simulink model "RadarSimulinkProjectRev009"  (R2024a)
settings: Solver=VariableStepAuto  StartTime=0.0  StopTime=0.0125  RelTol=1e-3
values from neighbouring files (symbols this model uses):
  AngleTime = SweepTime/10    (= 10000)    [InitializationOfVariables.m]    (also in InitializationOfVariablesRev000.m; InitializationOfVariablesRev001.m; InitializationOfVariablesRev003.m = 2097152; InitializationOfVariablesRev004.m = 2097152)
  ASR_LUT = Rsamp-OffsetDelayR    [InitializationOfVariablesRev003.m]    (also in InitializationOfVariablesRev004.m = round((R*2*SystemFs)/c))
  Btn_Debounce = 20000    [InitializationOfVariablesRev003.m]    (also in InitializationOfVariablesRev004.m)
  ChirpNc = 128    [InitializationOfVariablesRev003.m]    (also in InitializationOfVariablesRev004.m)
  ChirpSizeLength = FreqDeltaPeriod*361    (= 16245)    [InitializationOfVariablesRev003.m]    (also in InitializationOfVariablesRev004.m = 16384)
  DeciFactor = 8    [InitializationOfVariablesRev004.m]
  FCW = [FCW_p1, FCW_p2]    [InitializationOfVariablesRev003.m]    (also in InitializationOfVariablesRev004.m = f / SystemFs)
  RXFFTLength = 16384    [InitializationOfVariablesRev003.m]    (also in InitializationOfVariablesRev004.m = 2048)
  SweepTime = 100000    [InitializationOfVariables.m]    (also in InitializationOfVariablesRev000.m; InitializationOfVariablesRev001.m; InitializationOfVariablesRev003.m = 23068672; InitializationOfVariablesRev004.m = 23068672)
undefined symbols (not defined in the file or in its folder): SignalGenerationForAnalysis, Subsystem, xc7a200tfbg676
libraries: hdlBasic x407, hdlUtilities x11, hdlDSPIP x11, vmcUtilities x1
(part 3 of 4)

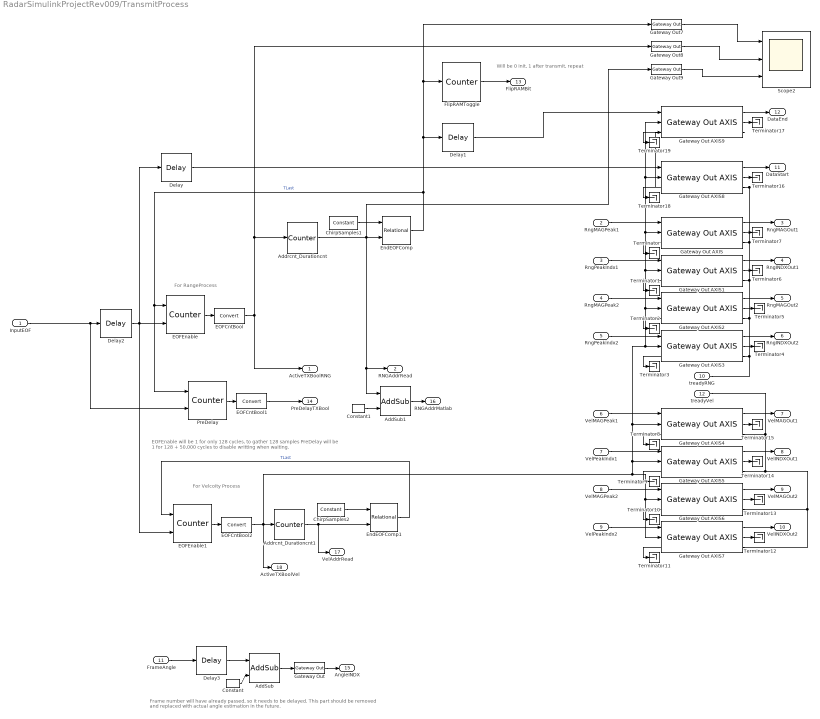
== system RadarSimulinkProjectRev009/TransmitProcess ==
  note: For RangeProcess
  note: Frame number will have already passed, so it needs to be delayed. This part should be removed and replaced with actual angle estimation in the future.
  note: EOFEnable will be 1 for only 128 cycles, to gather 128 samples
      | PreDelay will be 1 for 128 + 50,000 cycles to disable writting when waiting.
  note: Will be 0 init, 1 after transmit, repeat
  note: For Velcoity Process
  InputEOF : Inport
  RngMAGPeak1 : Inport  Port=2
  RngPeakIndx1 : Inport  Port=3
  RngMAGPeak2 : Inport  Port=4
  RngPeakindx2 : Inport  Port=5
  VelMAGPeak1 : Inport  Port=6
  VelPeakIndx1 : Inport  Port=7
  VelMAGPeak2 : Inport  Port=8
  VelPeakindx2 : Inport  Port=9
  treadyRNG : Inport  Port=10
  FrameAngle : Inport  Port=11
  treadyVel : Inport  Port=12
  AddSub : hdlBasic/AddSub  mode=Addition  use_carryin=off  use_carryout=off  en=off  latency=1  precision=Full  arith_type=Unsigned  n_bits=16  bin_pt=14  quantization=Truncate  overflow=Wrap  use_behavioral_HDL=off  hw_selection=Fabric  pipelined=off  XmcBlockStatus=1  maskContainerNames=tabcontainer1  block_type=addsub  block_config=sysgen:Addsub_config
  AddSub1 : hdlBasic/AddSub  mode=Addition  use_carryin=off  use_carryout=off  en=off  latency=1  precision=Full  arith_type=Unsigned  n_bits=16  bin_pt=14  quantization=Truncate  overflow=Wrap  use_behavioral_HDL=off  hw_selection=Fabric  pipelined=off  XmcBlockStatus=1  maskContainerNames=tabcontainer1  block_type=addsub  block_config=sysgen:Addsub_config
  Addrcnt_Durationcnt : hdlBasic/Counter  cnt_type=Count limited  cnt_to=ChirpNc-1  operation=Up  start_count=0  cnt_by_val=1  arith_type=Unsigned  n_bits=7  bin_pt=0  load_pin=off  rst=off  en=on  explicit_period=Explicit  period=P1  use_behavioral_HDL=off  implementation=Fabric  XmcBlockStatus=1  maskContainerNames=group1  block_type=counter  block_config=sysgen:Counter_config  block_width=531  block_height=1023
  Addrcnt_Durationcnt1 : hdlBasic/Counter  cnt_type=Count limited  cnt_to=RXFFTLength-1  operation=Up  start_count=0  cnt_by_val=1  arith_type=Unsigned  n_bits=11  bin_pt=0  load_pin=off  rst=off  en=on  explicit_period=Explicit  period=P1  use_behavioral_HDL=off  implementation=Fabric  XmcBlockStatus=1  maskContainerNames=group1  block_type=counter  block_config=sysgen:Counter_config  block_width=531  block_height=1023
  ChirpSamples1 : hdlBasic/Constant  const=127  gui_display_data_type=Fixed-point  arith_type=Unsigned  n_bits=7  bin_pt=0  preci_type=Single  exp_width=8  frac_width=24  explicit_period=on  period=P2  XmcBlockStatus=1  maskContainerNames=tabcontainer1  block_type=constant  block_config=sysgen:Constant_config
  ChirpSamples2 : hdlBasic/Constant  const=2047  gui_display_data_type=Fixed-point  arith_type=Unsigned  n_bits=15  bin_pt=0  preci_type=Single  exp_width=8  frac_width=24  explicit_period=on  period=P2  XmcBlockStatus=1  maskContainerNames=tabcontainer1  block_type=constant  block_config=sysgen:Constant_config
  Constant : hdlBasic/Constant  const=1.0  gui_display_data_type=Fixed-point  arith_type=Unsigned  n_bits=7  bin_pt=0  preci_type=Single  exp_width=8  frac_width=24  explicit_period=off  period=1  XmcBlockStatus=1  maskContainerNames=tabcontainer1  block_type=constant  block_config=sysgen:Constant_config
  Constant1 : hdlBasic/Constant  const=1.0  gui_display_data_type=Fixed-point  arith_type=Unsigned  n_bits=7  bin_pt=0  preci_type=Single  exp_width=8  frac_width=24  explicit_period=off  period=1  XmcBlockStatus=1  maskContainerNames=tabcontainer1  block_type=constant  block_config=sysgen:Constant_config
  Delay : hdlBasic/Delay  rst=off  en=off  latency=1  reg_retiming=off  XmcBlockStatus=1  maskContainerNames=group1  block_type=delay  block_config=sysgen:Delay_config
  Delay1 : hdlBasic/Delay  rst=off  en=off  latency=1  reg_retiming=off  XmcBlockStatus=1  maskContainerNames=group1  block_type=delay  block_config=sysgen:Delay_config
  Delay2 : hdlBasic/Delay  rst=off  en=off  latency=50000  reg_retiming=off  XmcBlockStatus=1  maskContainerNames=group1  block_type=delay  block_config=sysgen:Delay_config
  Delay3 : hdlBasic/Delay  rst=off  en=off  latency=64000  reg_retiming=off  XmcBlockStatus=1  maskContainerNames=group1  block_type=delay  block_config=sysgen:Delay_config
  EOFCntBool : hdlBasic/Convert  gui_display_data_type=Boolean  arith_type=Boolean  n_bits=16  bin_pt=14  float_type=Single  exp_bits=8  fraction_bits=24  quantization=Truncate  overflow=Wrap  en=off  latency=0  pipeline=off  XmcBlockStatus=1  maskContainerNames=group2  block_type=convert  block_config=sysgen:Convert_config  block_width=595  block_height=885
  EOFCntBool1 : hdlBasic/Convert  gui_display_data_type=Boolean  arith_type=Boolean  n_bits=16  bin_pt=14  float_type=Single  exp_bits=8  fraction_bits=24  quantization=Truncate  overflow=Wrap  en=off  latency=0  pipeline=off  XmcBlockStatus=1  maskContainerNames=group2  block_type=convert  block_config=sysgen:Convert_config  block_width=595  block_height=885
  EOFCntBool2 : hdlBasic/Convert  gui_display_data_type=Boolean  arith_type=Boolean  n_bits=16  bin_pt=14  float_type=Single  exp_bits=8  fraction_bits=24  quantization=Truncate  overflow=Wrap  en=off  latency=0  pipeline=off  XmcBlockStatus=1  maskContainerNames=group2  block_type=convert  block_config=sysgen:Convert_config  block_width=595  block_height=885
  EOFEnable : hdlBasic/Counter  cnt_type=Count limited  cnt_to=1  operation=Up  start_count=0  cnt_by_val=1  arith_type=Unsigned  n_bits=1  bin_pt=0  load_pin=off  rst=on  en=on  explicit_period=Explicit  period=P1  use_behavioral_HDL=off  implementation=Fabric  XmcBlockStatus=1  maskContainerNames=group1  block_type=counter  block_config=sysgen:Counter_config  block_width=531  block_height=1023
  EOFEnable1 : hdlBasic/Counter  cnt_type=Count limited  cnt_to=1  operation=Up  start_count=0  cnt_by_val=1  arith_type=Unsigned  n_bits=1  bin_pt=0  load_pin=off  rst=on  en=on  explicit_period=Explicit  period=P1  use_behavioral_HDL=off  implementation=Fabric  XmcBlockStatus=1  maskContainerNames=group1  block_type=counter  block_config=sysgen:Counter_config  block_width=531  block_height=1023
  EndEOFComp : hdlBasic/Relational  mode=a=b  op_type=Bool  en=off  latency=0  XmcBlockStatus=1  maskContainerNames=tabcontainer1  block_type=relational  block_config=sysgen:Relational_config
  EndEOFComp1 : hdlBasic/Relational  mode=a=b  op_type=Bool  en=off  latency=0  XmcBlockStatus=1  maskContainerNames=tabcontainer1  block_type=relational  block_config=sysgen:Relational_config
  FlipRAMToggle : hdlBasic/Counter  cnt_type=Count limited  cnt_to=1  operation=Up  start_count=0  cnt_by_val=1  arith_type=Unsigned  n_bits=1  bin_pt=0  load_pin=off  rst=off  en=on  explicit_period=Explicit  period=P1  use_behavioral_HDL=off  implementation=Fabric  XmcBlockStatus=1  maskContainerNames=group1  block_type=counter  block_config=sysgen:Counter_config  block_width=531  block_height=1023
  Gateway Out{,7..9} (4 alike) : hdlBasic/Gateway Out  inherit_from_input=off  bool_to_boolean=off  hdl_port=on  rows=1  columns=1  UseAsDAC=off  DACChannel='1'  interface=None  automatic_assignment=on  address_offset=hex2dec('00')  intf_name=''  intf_description=''  timing_constraint=None  locs_specified=off  LOCs={}  io_standard={}  XmcBlockStatus=1  maskContainerNames=group4  block_type=gatewayout  block_config=sysgen:gateway_out_config  block_width_w=590  block_height_w=620  block_width=620  block_height=750
  Gateway Out AXIS{,1..9} (10 alike) : hdlUtilities/Gateway Out AXIS  mask_sample_period=1  bool_to_boolean=off  block_type=gatewayoutaxi
  PreDelay : hdlBasic/Counter  cnt_type=Count limited  cnt_to=1  operation=Up  start_count=0  cnt_by_val=1  arith_type=Unsigned  n_bits=1  bin_pt=0  load_pin=off  rst=on  en=on  explicit_period=Explicit  period=P1  use_behavioral_HDL=off  implementation=Fabric  XmcBlockStatus=1  maskContainerNames=group1  block_type=counter  block_config=sysgen:Counter_config  block_width=531  block_height=1023
  Scope2 : Scope  NumInputPorts=3
  Terminator{,1..19} (20 alike) : Terminator
  ActiveTXBoolRNG : Outport
  RNGAddrRead : Outport  Port=2
  RngMAGOut1 : Outport  Port=3
  RngINDXOut1 : Outport  Port=4
  RngMAGOut2 : Outport  Port=5
  RngINDXOut2 : Outport  Port=6
  VelMAGOut1 : Outport  Port=7
  VelINDXOut1 : Outport  Port=8
  VelMAGOut2 : Outport  Port=9
  VelINDXOut2 : Outport  Port=10
  DataStart : Outport  Port=11
  DataEnd : Outport  Port=12
  FlipRAMBit : Outport  Port=13
  PreDelayTXBool : Outport  Port=14
  AngleINDX : Outport  Port=15
  RNGAddrMatlab : Outport  Port=16
  VelAddrRead : Outport  Port=17
  ActiveTXBoolVel : Outport  Port=18
  wires:
  ChirpSamples1/1 -> EndEOFComp/1
  Gateway Out AXIS/1 -> RngMAGOut1/1
  Gateway Out AXIS2/3 -> Terminator2/1
  Gateway Out AXIS3/1 -> RngINDXOut2/1
  Gateway Out AXIS1/3 -> Terminator1/1
  Gateway Out AXIS1/1 -> RngINDXOut1/1
  Gateway Out AXIS/2 -> Terminator7/1
  EndEOFComp/1 -> Gateway Out7/1, FlipRAMToggle/1, Delay1/1, PreDelay/1, EOFEnable/1  "TLast"
  Gateway Out AXIS2/1 -> RngMAGOut2/1
  EOFEnable/1 -> EOFCntBool/1
  RngMAGPeak2/1 -> Gateway Out AXIS2/1
  Gateway Out AXIS2/2 -> Terminator5/1
  RngPeakIndx1/1 -> Gateway Out AXIS1/1
  RngMAGPeak1/1 -> Gateway Out AXIS/1
  Gateway Out AXIS1/2 -> Terminator6/1
  RngPeakindx2/1 -> Gateway Out AXIS3/1
  Gateway Out AXIS3/3 -> Terminator3/1
  Gateway Out AXIS3/2 -> Terminator4/1
  Gateway Out AXIS/3 -> Terminator/1
  Gateway Out AXIS7/3 -> Terminator11/1
  VelPeakindx2/1 -> Gateway Out AXIS7/1
  Gateway Out AXIS6/3 -> Terminator10/1
  VelMAGPeak2/1 -> Gateway Out AXIS6/1
  Gateway Out AXIS5/2 -> Terminator14/1
  Gateway Out AXIS6/1 -> VelMAGOut2/1
  Gateway Out AXIS7/1 -> VelINDXOut2/1
  Gateway Out AXIS5/1 -> VelINDXOut1/1
  EOFCntBool/1 -> Gateway Out8/1, Addrcnt_Durationcnt/1, ActiveTXBoolRNG/1
  VelPeakIndx1/1 -> Gateway Out AXIS5/1
  Gateway Out AXIS4/3 -> Terminator8/1
  Gateway Out AXIS6/2 -> Terminator13/1
  VelMAGPeak1/1 -> Gateway Out AXIS4/1
  Gateway Out AXIS7/2 -> Terminator12/1
  Gateway Out AXIS4/1 -> VelMAGOut1/1
  Gateway Out AXIS5/3 -> Terminator9/1
  Gateway Out AXIS4/2 -> Terminator15/1
  treadyRNG/1 -> Gateway Out AXIS9/3, Gateway Out AXIS8/3, Gateway Out AXIS/3, Gateway Out AXIS1/3, Gateway Out AXIS2/3, Gateway Out AXIS3/3
  Gateway Out AXIS8/1 -> DataStart/1
  Gateway Out AXIS8/2 -> Terminator16/1
  Gateway Out AXIS9/1 -> DataEnd/1
  Gateway Out AXIS9/2 -> Terminator17/1
  Gateway Out AXIS8/3 -> Terminator18/1
  Gateway Out AXIS9/3 -> Terminator19/1
  Delay/1 -> Gateway Out AXIS8/1
  Delay1/1 -> Gateway Out AXIS9/1
  Delay2/1 -> EOFEnable1/2, Delay/1, EOFEnable/2
  FlipRAMToggle/1 -> FlipRAMBit/1
  PreDelay/1 -> EOFCntBool1/1
  EOFCntBool1/1 -> PreDelayTXBool/1
  FrameAngle/1 -> Delay3/1
  Delay3/1 -> AddSub/1
  Gateway Out/1 -> AngleINDX/1
  Constant/1 -> AddSub/2
  AddSub/1 -> Gateway Out/1
  Addrcnt_Durationcnt/1 -> Gateway Out9/1, EndEOFComp/2, RNGAddrRead/1, AddSub1/1
  AddSub1/1 -> RNGAddrMatlab/1
  Constant1/1 -> AddSub1/2
  InputEOF/1 -> PreDelay/2, Delay2/1
  Addrcnt_Durationcnt1/1 -> VelAddrRead/1, EndEOFComp1/2
  ChirpSamples2/1 -> EndEOFComp1/1
  EndEOFComp1/1 -> EOFEnable1/1  "TLast"
  EOFEnable1/1 -> EOFCntBool2/1
  EOFCntBool2/1 -> ActiveTXBoolVel/1, Gateway Out AXIS4/2, Gateway Out AXIS3/2, Gateway Out AXIS9/2, Gateway Out AXIS8/2, Gateway Out AXIS/2, Gateway Out AXIS1/2, Gateway Out AXIS2/2, Gateway Out AXIS5/2, Gateway Out AXIS6/2, Gateway Out AXIS7/2, Addrcnt_Durationcnt1/1
  treadyVel/1 -> Gateway Out AXIS7/3, Gateway Out AXIS6/3, Gateway Out AXIS5/3, Gateway Out AXIS4/3
  Gateway Out8/1 -> Scope2/2
  Gateway Out9/1 -> Scope2/3
  Gateway Out7/1 -> Scope2/1

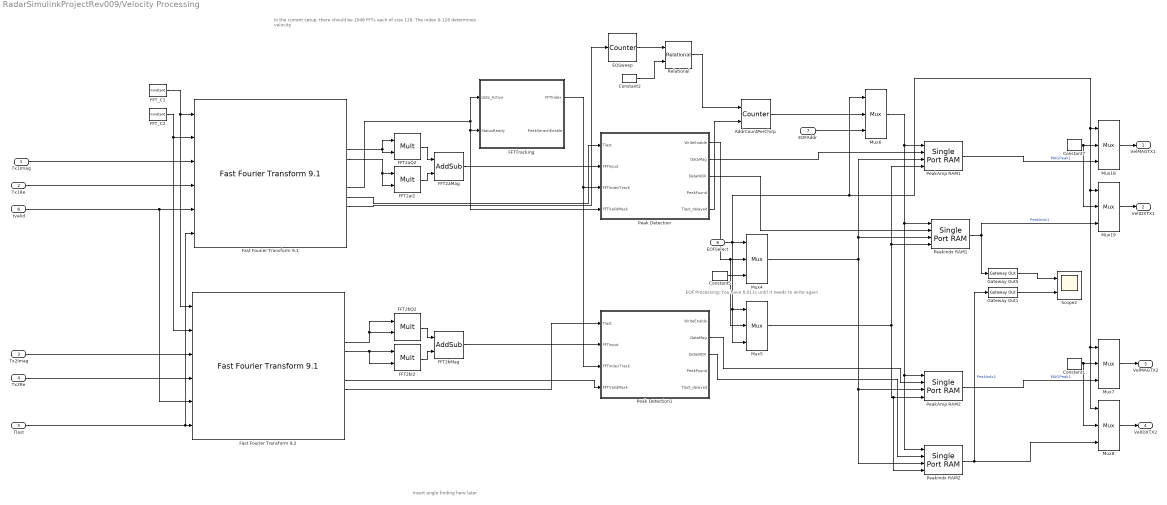
== system RadarSimulinkProjectRev009/Velocity Processing ==
  note: In the current setup, there should be 2048 FFTs each of size 128. The index 0-128 determines velocity
  note: EOF Processing: You have 0.011s until it needs to write again
  note: Insert angle finding here later
  Tx1Imag : Inport
  Tx1Re : Inport  Port=2
  Tx2Imag : Inport  Port=3
  Tx2Re : Inport  Port=4
  Tlast : Inport  Port=5
  tvalid : Inport  Port=6
  EOFAddr : Inport  Port=7
  EOFSelect : Inport  Port=8
  AddrCountPerChirp : hdlBasic/Counter  cnt_type=Count limited  cnt_to=RXFFTLength-1  operation=Up  start_count=0  cnt_by_val=1  arith_type=Unsigned  n_bits=11  bin_pt=0  load_pin=off  rst=on  en=on  explicit_period=Explicit  period=P1  use_behavioral_HDL=off  implementation=Fabric  XmcBlockStatus=1  maskContainerNames=group1  block_type=counter  block_config=sysgen:Counter_config  block_width=531  block_height=1023
  Constant1 : hdlBasic/Constant  const=0  gui_display_data_type=Fixed-point  arith_type=Signed (2's comp)  n_bits=16  bin_pt=15  preci_type=Single  exp_width=8  frac_width=24  explicit_period=on  period=P2  XmcBlockStatus=1  maskContainerNames=tabcontainer1  block_type=constant  block_config=sysgen:Constant_config
  Constant2 : hdlBasic/Constant  const=0  gui_display_data_type=Fixed-point  arith_type=Signed (2's comp)  n_bits=1  bin_pt=0  preci_type=Single  exp_width=8  frac_width=24  explicit_period=on  period=P1  XmcBlockStatus=1  maskContainerNames=tabcontainer1  block_type=constant  block_config=sysgen:Constant_config
  Constant5 : hdlBasic/Constant  const=0  gui_display_data_type=Boolean  arith_type=Boolean  n_bits=16  bin_pt=15  preci_type=Single  exp_width=8  frac_width=24  explicit_period=on  period=P2  XmcBlockStatus=1  maskContainerNames=tabcontainer1  block_type=constant  block_config=sysgen:Constant_config
  Constant7 : hdlBasic/Constant  const=0  gui_display_data_type=Fixed-point  arith_type=Signed (2's comp)  n_bits=16  bin_pt=15  preci_type=Single  exp_width=8  frac_width=24  explicit_period=on  period=P2  XmcBlockStatus=1  maskContainerNames=tabcontainer1  block_type=constant  block_config=sysgen:Constant_config
  EOSweep : hdlBasic/Counter  cnt_type=Count limited  cnt_to=ChirpNc*11-1  operation=Up  start_count=0  cnt_by_val=1  arith_type=Unsigned  n_bits=11  bin_pt=0  load_pin=off  rst=off  en=on  explicit_period=Explicit  period=P1  use_behavioral_HDL=off  implementation=Fabric  XmcBlockStatus=1  maskContainerNames=group1  block_type=counter  block_config=sysgen:Counter_config  block_width=531  block_height=1023
  FFT2aI2 : hdlBasic/Mult  precision=Full  arith_type="Signed  (2's comp)"  n_bits=16  bin_pt=14  quantization=Truncate  overflow=Wrap  en=off  latency=3  opt_float=off  fp_mult_usage=No Usage  use_behavioral_HDL=off  opt=Speed  use_embedded=on  optimum_pipeline=off  pipeline=on  use_rpm=on  placement_style=Triangular  XmcBlockStatus=1  maskContainerNames=group1  block_type=mult  block_config=sysgen:Mult_config  block_width=598  block_height=876
  FFT2aMag : hdlBasic/AddSub  mode=Addition  use_carryin=off  use_carryout=off  en=off  latency=0  precision=Full  arith_type=Unsigned  n_bits=16  bin_pt=14  quantization=Truncate  overflow=Wrap  use_behavioral_HDL=off  hw_selection=Fabric  pipelined=off  XmcBlockStatus=1  maskContainerNames=tabcontainer1  block_type=addsub  block_config=sysgen:Addsub_config
  FFT2aQ2 : hdlBasic/Mult  precision=Full  arith_type="Signed  (2's comp)"  n_bits=16  bin_pt=14  quantization=Truncate  overflow=Wrap  en=off  latency=3  opt_float=off  fp_mult_usage=No Usage  use_behavioral_HDL=off  opt=Speed  use_embedded=on  optimum_pipeline=off  pipeline=on  use_rpm=on  placement_style=Triangular  XmcBlockStatus=1  maskContainerNames=group1  block_type=mult  block_config=sysgen:Mult_config  block_width=598  block_height=876
  FFT2bI2 : hdlBasic/Mult  precision=Full  arith_type="Signed  (2's comp)"  n_bits=16  bin_pt=14  quantization=Truncate  overflow=Wrap  en=off  latency=3  opt_float=off  fp_mult_usage=No Usage  use_behavioral_HDL=off  opt=Speed  use_embedded=on  optimum_pipeline=off  pipeline=on  use_rpm=on  placement_style=Triangular  XmcBlockStatus=1  maskContainerNames=group1  block_type=mult  block_config=sysgen:Mult_config  block_width=598  block_height=876
  FFT2bMag : hdlBasic/AddSub  mode=Addition  use_carryin=off  use_carryout=off  en=off  latency=0  precision=Full  arith_type=Unsigned  n_bits=16  bin_pt=14  quantization=Truncate  overflow=Wrap  use_behavioral_HDL=off  hw_selection=Fabric  pipelined=off  XmcBlockStatus=1  maskContainerNames=tabcontainer1  block_type=addsub  block_config=sysgen:Addsub_config
  FFT2bQ2 : hdlBasic/Mult  precision=Full  arith_type="Signed  (2's comp)"  n_bits=16  bin_pt=14  quantization=Truncate  overflow=Wrap  en=off  latency=3  opt_float=off  fp_mult_usage=No Usage  use_behavioral_HDL=off  opt=Speed  use_embedded=on  optimum_pipeline=off  pipeline=on  use_rpm=on  placement_style=Triangular  XmcBlockStatus=1  maskContainerNames=group1  block_type=mult  block_config=sysgen:Mult_config  block_width=598  block_height=876
  FFTTracking : Subsystem
  FFT_C1 : hdlBasic/Constant  const=1.0  gui_display_data_type=Fixed-point  arith_type=Unsigned  n_bits=1  bin_pt=0  preci_type=Single  exp_width=8  frac_width=24  explicit_period=on  period=P2  XmcBlockStatus=1  maskContainerNames=tabcontainer1  block_type=constant  block_config=sysgen:Constant_config
  FFT_C2 : hdlBasic/Constant  const=1.0  gui_display_data_type=Boolean  arith_type=Boolean  n_bits=1  bin_pt=0  preci_type=Single  exp_width=8  frac_width=24  explicit_period=on  period=P2  XmcBlockStatus=1  maskContainerNames=tabcontainer1  block_type=constant  block_config=sysgen:Constant_config
  Fast Fourier Transform 9.1 : hdlDSPIP/Fast Fourier Transform 9.1   transform_length=128  target_clock_frequency=192  target_data_throughput=50  implementation_options=pipelined_streaming_io  run_time_configurable_transform_length=off  enable_ssr=off  super_sample_rates=1  data_format=fixed_point  phase_factor_width=32  scaling_options=block_floating_point  rounding_modes=truncation  aclken=off  aresetn=off  output_ordering=natural_order  cyclic_prefix_insertion=off  throttle_scheme=realtime  xk_index=on  ovflo=off  trim_axipin_name=on  memory_options_data=block_ram  memory_options_phase_factors=block_ram  number_of_stages_using_block_ram_for_data_and_phase_factors=2  memory_options_reorder=block_ram  memory_options_hybrid=off  complex_mult_type=use_mults_resources  butterfly_type=use_xtremedsp_slices  simulation_type=hybrid_sim  simulation_model=sysgen:xfftv9_cmodel  data_path_portlist={ 's_axis_data_tdata', 'm_axis_data_tdata', 'm_axis_status_tdata', 'event_fft_overflow' }  channels=1  input_ordering=natural_order  input_width=16  ip_name=Fast Fourier Transform  ip_version=9.1  dsptool_ready=true  ipcore_usecache=true  ipcore_useipmodelcache=true  wrapper_available=true  port_translation_map={ 'aclken' => 'en', 'aresetn' => 'rst'}  XmcBlockStatus=1  maskContainerNames=tabcontainer1  block_type=xfft_v9_1  block_config=sysgen:rodinimport_config
  Fast Fourier Transform 9.2 : hdlDSPIP/Fast Fourier Transform 9.1   transform_length=128  target_clock_frequency=192  target_data_throughput=50  implementation_options=pipelined_streaming_io  run_time_configurable_transform_length=off  enable_ssr=off  super_sample_rates=1  data_format=fixed_point  phase_factor_width=32  scaling_options=block_floating_point  rounding_modes=truncation  aclken=off  aresetn=off  output_ordering=natural_order  cyclic_prefix_insertion=off  throttle_scheme=realtime  xk_index=on  ovflo=off  trim_axipin_name=on  memory_options_data=block_ram  memory_options_phase_factors=block_ram  number_of_stages_using_block_ram_for_data_and_phase_factors=2  memory_options_reorder=block_ram  memory_options_hybrid=off  complex_mult_type=use_mults_resources  butterfly_type=use_xtremedsp_slices  simulation_type=hybrid_sim  simulation_model=sysgen:xfftv9_cmodel  data_path_portlist={ 's_axis_data_tdata', 'm_axis_data_tdata', 'm_axis_status_tdata', 'event_fft_overflow' }  channels=1  input_ordering=natural_order  input_width=16  ip_name=Fast Fourier Transform  ip_version=9.1  dsptool_ready=true  ipcore_usecache=true  ipcore_useipmodelcache=true  wrapper_available=true  port_translation_map={ 'aclken' => 'en', 'aresetn' => 'rst'}  XmcBlockStatus=1  maskContainerNames=tabcontainer1  block_type=xfft_v9_1  block_config=sysgen:rodinimport_config
  Gateway Out1 : hdlBasic/Gateway Out  inherit_from_input=off  bool_to_boolean=off  hdl_port=on  rows=1  columns=1  UseAsDAC=off  DACChannel='1'  interface=None  automatic_assignment=on  address_offset=hex2dec('00')  intf_name=''  intf_description=''  timing_constraint=None  locs_specified=off  LOCs={}  io_standard={}  XmcBlockStatus=1  maskContainerNames=group4  block_type=gatewayout  block_config=sysgen:gateway_out_config  block_width_w=590  block_height_w=620  block_width=620  block_height=750
  Gateway Out5 : hdlBasic/Gateway Out  inherit_from_input=off  bool_to_boolean=off  hdl_port=on  rows=1  columns=1  UseAsDAC=off  DACChannel='1'  interface=None  automatic_assignment=on  address_offset=hex2dec('00')  intf_name=''  intf_description=''  timing_constraint=None  locs_specified=off  LOCs={}  io_standard={}  XmcBlockStatus=1  maskContainerNames=group4  block_type=gatewayout  block_config=sysgen:gateway_out_config  block_width_w=590  block_height_w=620  block_width=620  block_height=750
  Mux{4..8,18..19} (7 alike) : hdlBasic/Mux  inputs=2  en=off  latency=0  precision=Full  arith_type=Unsigned  n_bits=16  bin_pt=14  quantization=Truncate  overflow=Wrap  XmcBlockStatus=1  maskContainerNames=tabcontainer1  block_type=mux  block_config=sysgen:Mux_config
  Peak Detection : Subsystem
  Peak Detection1 : Subsystem
  PeakAmp RAM1 : hdlBasic/Single Port RAM  depth=RXFFTLength  initVector=0  distributed_mem=Block RAM  write_mode=Read After Write  rst=off  init_reg=0  en=on  optimize_latency=off  latency=1  optimize=Area  dbl_ovrd=off  simulation_type=fast_sim  XmcBlockStatus=1  maskContainerNames=tabcontainer1  block_type=spram  block_config=sysgen:SPRAM_config
  PeakAmp RAM2 : hdlBasic/Single Port RAM  depth=RXFFTLength  initVector=0  distributed_mem=Block RAM  write_mode=Read After Write  rst=off  init_reg=0  en=on  optimize_latency=off  latency=1  optimize=Area  dbl_ovrd=off  simulation_type=fast_sim  XmcBlockStatus=1  maskContainerNames=tabcontainer1  block_type=spram  block_config=sysgen:SPRAM_config
  PeakIndx RAM1 : hdlBasic/Single Port RAM  depth=RXFFTLength  initVector=0  distributed_mem=Block RAM  write_mode=Read After Write  rst=off  init_reg=0  en=on  optimize_latency=off  latency=1  optimize=Area  dbl_ovrd=off  simulation_type=fast_sim  XmcBlockStatus=1  maskContainerNames=tabcontainer1  block_type=spram  block_config=sysgen:SPRAM_config
  PeakIndx RAM2 : hdlBasic/Single Port RAM  depth=RXFFTLength  initVector=0  distributed_mem=Block RAM  write_mode=Read After Write  rst=off  init_reg=0  en=on  optimize_latency=off  latency=1  optimize=Area  dbl_ovrd=off  simulation_type=fast_sim  XmcBlockStatus=1  maskContainerNames=tabcontainer1  block_type=spram  block_config=sysgen:SPRAM_config
  Relational : hdlBasic/Relational  mode=a=b  op_type=Bool  en=off  latency=0  XmcBlockStatus=1  maskContainerNames=tabcontainer1  block_type=relational  block_config=sysgen:Relational_config
  Scope2 : Scope  NumInputPorts=2
  VelMAGTX1 : Outport
  VelIDXTX1 : Outport  Port=2
  VelMAGTX2 : Outport  Port=3
  VelIDXTX2 : Outport  Port=4
  wires:
  FFT_C1/1 -> Fast Fourier Transform 9.2/1, Fast Fourier Transform 9.1/1
  FFT_C2/1 -> Fast Fourier Transform 9.2/2, Fast Fourier Transform 9.1/2
  tvalid/1 -> Fast Fourier Transform 9.2/5, Fast Fourier Transform 9.1/5
  Tx1Imag/1 -> Fast Fourier Transform 9.1/3
  Tlast/1 -> Fast Fourier Transform 9.1/6, Fast Fourier Transform 9.2/6
  Fast Fourier Transform 9.1/5 -> FFT2aQ2/1, FFT2aQ2/2
  FFT2aI2/1 -> FFT2aMag/2
  FFT2aQ2/1 -> FFT2aMag/1
  Fast Fourier Transform 9.1/6 -> FFT2aI2/2, FFT2aI2/1
  Fast Fourier Transform 9.1/9 -> FFTTracking/1(data_Active), FFTTracking/2(StatusReady), Peak Detection/4(FFTValidMask)
  FFT2bI2/1 -> FFT2bMag/2
  FFT2bQ2/1 -> FFT2bMag/1
  Constant5/1 -> Mux4/3
  Mux4/1 -> PeakIndx RAM1/3, PeakAmp RAM1/3, PeakIndx RAM2/3, PeakAmp RAM2/3
  Mux5/1 -> PeakIndx RAM2/4, PeakAmp RAM2/4, PeakAmp RAM1/4, PeakIndx RAM1/4
  PeakAmp RAM1/1 -> Mux18/3  "MAGPeak1"
  Mux6/1 -> PeakIndx RAM2/1, PeakAmp RAM2/1, PeakIndx RAM1/1, PeakAmp RAM1/1
  PeakIndx RAM1/1 -> Mux19/3, Gateway Out5/1  "PeakIndx1"
  PeakAmp RAM2/1 -> Mux7/3  "MAGPeak1"
  PeakIndx RAM2/1 -> Gateway Out1/1, Mux8/3  "PeakIndx1"
  Mux18/1 -> VelMAGTX1/1
  Mux19/1 -> VelIDXTX1/1
  Constant7/1 -> Mux19/2, Mux18/2
  Mux8/1 -> VelIDXTX2/1
  Mux7/1 -> VelMAGTX2/1
  EOFSelect/1 -> Mux6/1, Mux7/1, Mux8/1, Mux19/1, Mux18/1, Mux5/3, Mux5/1, Mux4/1
  Constant1/1 -> Mux8/2, Mux7/2
  EOFAddr/1 -> Mux6/3
  Fast Fourier Transform 9.2/6 -> FFT2bI2/1, FFT2bI2/2
  AddrCountPerChirp/1 -> Mux6/2
  Fast Fourier Transform 9.2/5 -> FFT2bQ2/1, FFT2bQ2/2
  Gateway Out5/1 -> Scope2/1
  Tx1Re/1 -> Fast Fourier Transform 9.1/4
  FFT2aMag/1 -> Peak Detection/2(FFTInput)
  FFTTracking/1(FFTIndex) -> Peak Detection1/3(FFTIndexTrack), Peak Detection/3(FFTIndexTrack)
  Fast Fourier Transform 9.1/10 -> Peak Detection/1(Tlast)
  Peak Detection/1(WriteEnable) -> Mux5/2, Mux4/2
  Peak Detection/2(DataMag) -> PeakAmp RAM1/2
  Peak Detection/3(DataINDX) -> PeakIndx RAM1/2
  Peak Detection/5(Tlast_delayed) -> AddrCountPerChirp/2
  Fast Fourier Transform 9.1/11 -> EOSweep/1
  EOSweep/1 -> Relational/1
  Constant2/1 -> Relational/2
  Relational/1 -> AddrCountPerChirp/1
  Fast Fourier Transform 9.2/10 -> Peak Detection1/1(Tlast)
  FFT2bMag/1 -> Peak Detection1/2(FFTInput)
  Fast Fourier Transform 9.2/9 -> Peak Detection1/4(FFTValidMask)
  Peak Detection1/2(DataMag) -> PeakAmp RAM2/2
  Peak Detection1/3(DataINDX) -> PeakIndx RAM2/2
  Gateway Out1/1 -> Scope2/2
  Tx2Imag/1 -> Fast Fourier Transform 9.2/3
  Tx2Re/1 -> Fast Fourier Transform 9.2/4

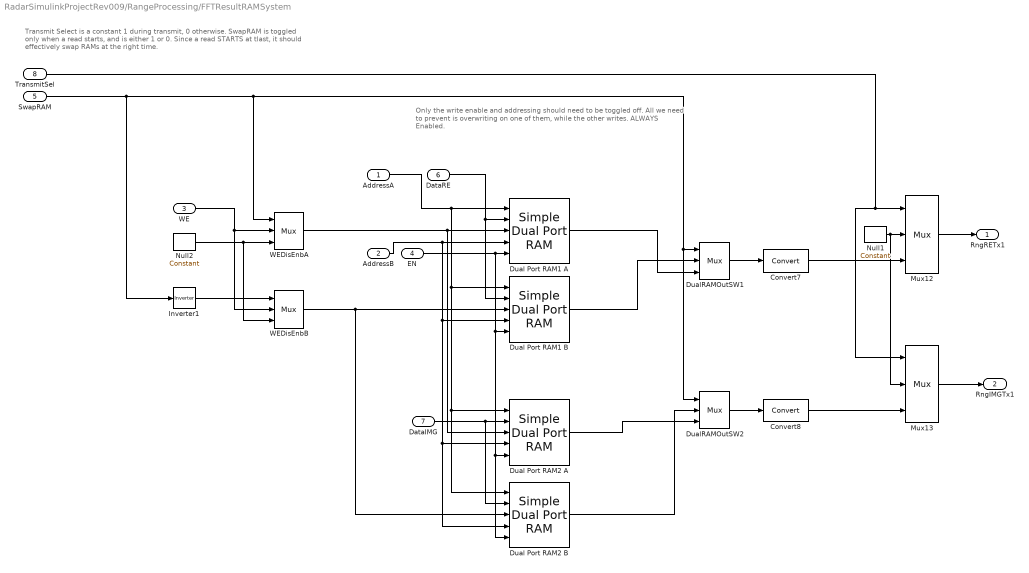
== system RadarSimulinkProjectRev009/RangeProcessing/FFTResultRAMSystem ==
  note: Transmit Select is a constant 1 during transmit, 0 otherwise.
      | SwapRAM is toggled only when a read starts, and is either 1 or 0.
      | Since a read STARTS at tlast, it should effectively swap RAMs at the right time.
  note: Only the write enable and addressing should need to be toggled off.
      | All we need to prevent is overwriting on one of them, while the other writes.
      | ALWAYS Enabled.
  AddressA : Inport
  AddressB : Inport  Port=2
  WE : Inport  Port=3
  EN : Inport  Port=4
  SwapRAM : Inport  Port=5
  DataRE : Inport  Port=6
  DataIMG : Inport  Port=7
  TransmitSel : Inport  Port=8
  Convert7 : hdlBasic/Convert  gui_display_data_type=Fixed-point  arith_type="Signed  (2's comp)"  n_bits=17  bin_pt=16  float_type=Single  exp_bits=8  fraction_bits=24  quantization=Truncate  overflow=Saturate  en=off  latency=0  pipeline=off  XmcBlockStatus=1  maskContainerNames=group2  block_type=convert  block_config=sysgen:Convert_config  block_width=595  block_height=885
  Convert8 : hdlBasic/Convert  gui_display_data_type=Fixed-point  arith_type="Signed  (2's comp)"  n_bits=17  bin_pt=16  float_type=Single  exp_bits=8  fraction_bits=24  quantization=Truncate  overflow=Saturate  en=off  latency=0  pipeline=off  XmcBlockStatus=1  maskContainerNames=group2  block_type=convert  block_config=sysgen:Convert_config  block_width=595  block_height=885
  Dual Port RAM1 A : hdlBasic/Simple Dual Port RAM  depth=ChirpNc*RXFFTLength  initVector=0  distributed_mem=Distributed memory  init_b=0  rst_b=off  en_a=on  en_b=off  latency=1  write_mode_B=Read After Write  explicit_period=[]  period=[]  simulation_type=fast_sim  XmcBlockStatus=1  maskContainerNames=tabcontainer1  block_type=sdpram  block_config=sysgen:Sdpram_config  optimize=Area
      settings: infoedit=[]
  Dual Port RAM1 B : hdlBasic/Simple Dual Port RAM  depth=ChirpNc*RXFFTLength  initVector=0  distributed_mem=Distributed memory  init_b=0  rst_b=off  en_a=on  en_b=off  latency=1  write_mode_B=Read After Write  explicit_period=[]  period=[]  simulation_type=fast_sim  XmcBlockStatus=1  maskContainerNames=tabcontainer1  block_type=sdpram  block_config=sysgen:Sdpram_config  optimize=Area
      settings: infoedit=[]
  Dual Port RAM2 A : hdlBasic/Simple Dual Port RAM  depth=ChirpNc*RXFFTLength  initVector=0  distributed_mem=Distributed memory  init_b=0  rst_b=off  en_a=on  en_b=off  latency=1  write_mode_B=Read After Write  explicit_period=[]  period=[]  simulation_type=fast_sim  XmcBlockStatus=1  maskContainerNames=tabcontainer1  block_type=sdpram  block_config=sysgen:Sdpram_config  optimize=Area
      settings: infoedit=[]
  Dual Port RAM2 B : hdlBasic/Simple Dual Port RAM  depth=ChirpNc*RXFFTLength  initVector=0  distributed_mem=Distributed memory  init_b=0  rst_b=off  en_a=on  en_b=off  latency=1  write_mode_B=Read After Write  explicit_period=[]  period=[]  simulation_type=fast_sim  XmcBlockStatus=1  maskContainerNames=tabcontainer1  block_type=sdpram  block_config=sysgen:Sdpram_config  optimize=Area
      settings: infoedit=[]
  DualRAMOutSW1 : hdlBasic/Mux  inputs=2  en=off  latency=0  precision=Full  arith_type=Unsigned  n_bits=16  bin_pt=14  quantization=Truncate  overflow=Wrap  XmcBlockStatus=1  maskContainerNames=tabcontainer1  block_type=mux  block_config=sysgen:Mux_config
  DualRAMOutSW2 : hdlBasic/Mux  inputs=2  en=off  latency=0  precision=Full  arith_type=Unsigned  n_bits=16  bin_pt=14  quantization=Truncate  overflow=Wrap  XmcBlockStatus=1  maskContainerNames=tabcontainer1  block_type=mux  block_config=sysgen:Mux_config
  Inverter1 : hdlBasic/Inverter  en=off  latency=0  XmcBlockStatus=1  maskContainerNames=group2  block_type=inv  block_config=sysgen:Inverter_config
  Mux12 : hdlBasic/Mux  inputs=2  en=off  latency=0  precision=Full  arith_type=Unsigned  n_bits=16  bin_pt=14  quantization=Truncate  overflow=Wrap  XmcBlockStatus=1  maskContainerNames=tabcontainer1  block_type=mux  block_config=sysgen:Mux_config
  Mux13 : hdlBasic/Mux  inputs=2  en=off  latency=0  precision=Full  arith_type=Unsigned  n_bits=16  bin_pt=14  quantization=Truncate  overflow=Wrap  XmcBlockStatus=1  maskContainerNames=tabcontainer1  block_type=mux  block_config=sysgen:Mux_config
  Null1 : hdlBasic/Constant  const=0  gui_display_data_type=Fixed-point  arith_type=Signed (2's comp)  n_bits=16  bin_pt=15  preci_type=Single  exp_width=8  frac_width=24  explicit_period=on  period=P2  XmcBlockStatus=1  maskContainerNames=tabcontainer1  block_type=constant  block_config=sysgen:Constant_config
  Null2 : hdlBasic/Constant  const=0  gui_display_data_type=Boolean  arith_type=Boolean  n_bits=16  bin_pt=15  preci_type=Single  exp_width=8  frac_width=24  explicit_period=on  period=P2  XmcBlockStatus=1  maskContainerNames=tabcontainer1  block_type=constant  block_config=sysgen:Constant_config
  WEDisEnbA : hdlBasic/Mux  inputs=2  en=off  latency=0  precision=Full  arith_type=Unsigned  n_bits=16  bin_pt=14  quantization=Truncate  overflow=Wrap  XmcBlockStatus=1  maskContainerNames=tabcontainer1  block_type=mux  block_config=sysgen:Mux_config
  WEDisEnbB : hdlBasic/Mux  inputs=2  en=off  latency=0  precision=Full  arith_type=Unsigned  n_bits=16  bin_pt=14  quantization=Truncate  overflow=Wrap  XmcBlockStatus=1  maskContainerNames=tabcontainer1  block_type=mux  block_config=sysgen:Mux_config
  RngRETx1 : Outport
  RngIMGTx1 : Outport  Port=2
  wires:
  Mux13/1 -> RngIMGTx1/1
  Mux12/1 -> RngRETx1/1
  Convert8/1 -> Mux13/3
  Convert7/1 -> Mux12/3
  TransmitSel/1 -> Mux12/1, Mux13/1
  Dual Port RAM2 A/1 -> DualRAMOutSW2/3
  Dual Port RAM1 A/1 -> DualRAMOutSW1/3
  Null1/1 -> Mux13/2, Mux12/2
  Dual Port RAM1 B/1 -> DualRAMOutSW1/2
  DualRAMOutSW1/1 -> Convert7/1
  DataRE/1 -> Dual Port RAM1 B/2, Dual Port RAM1 A/2
  DataIMG/1 -> Dual Port RAM2 B/2, Dual Port RAM2 A/2
  EN/1 -> Dual Port RAM1 A/5, Dual Port RAM1 B/5, Dual Port RAM2 B/5, Dual Port RAM2 A/5
  Null2/1 -> WEDisEnbB/3, WEDisEnbA/3
  Dual Port RAM2 B/1 -> DualRAMOutSW2/2
  DualRAMOutSW2/1 -> Convert8/1
  WE/1 -> WEDisEnbB/2, WEDisEnbA/2
  AddressA/1 -> Dual Port RAM1 A/1, Dual Port RAM1 B/1, Dual Port RAM2 A/1, Dual Port RAM2 B/1
  AddressB/1 -> Dual Port RAM2 A/4, Dual Port RAM2 B/4, Dual Port RAM1 B/4, Dual Port RAM1 A/4
  Inverter1/1 -> WEDisEnbB/1
  SwapRAM/1 -> Inverter1/1, WEDisEnbA/1, DualRAMOutSW2/1, DualRAMOutSW1/1
  WEDisEnbA/1 -> Dual Port RAM2 A/3, Dual Port RAM1 A/3
  WEDisEnbB/1 -> Dual Port RAM2 B/3, Dual Port RAM1 B/3

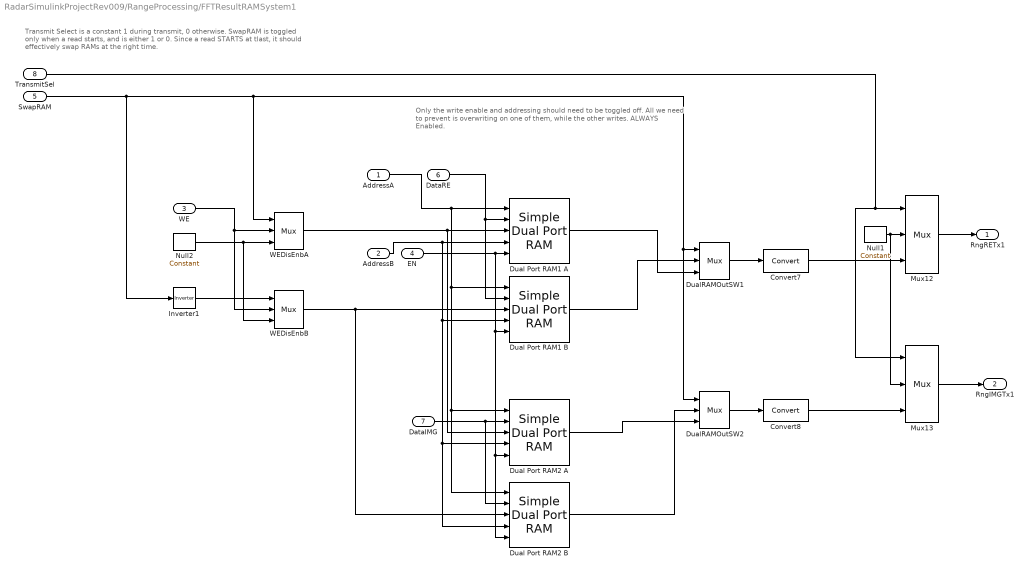
== system RadarSimulinkProjectRev009/RangeProcessing/FFTResultRAMSystem1 ==
  note: Transmit Select is a constant 1 during transmit, 0 otherwise.
      | SwapRAM is toggled only when a read starts, and is either 1 or 0.
      | Since a read STARTS at tlast, it should effectively swap RAMs at the right time.
  note: Only the write enable and addressing should need to be toggled off.
      | All we need to prevent is overwriting on one of them, while the other writes.
      | ALWAYS Enabled.
  AddressA : Inport
  AddressB : Inport  Port=2
  WE : Inport  Port=3
  EN : Inport  Port=4
  SwapRAM : Inport  Port=5
  DataRE : Inport  Port=6
  DataIMG : Inport  Port=7
  TransmitSel : Inport  Port=8
  Convert7 : hdlBasic/Convert  gui_display_data_type=Fixed-point  arith_type="Signed  (2's comp)"  n_bits=17  bin_pt=16  float_type=Single  exp_bits=8  fraction_bits=24  quantization=Truncate  overflow=Saturate  en=off  latency=0  pipeline=off  XmcBlockStatus=1  maskContainerNames=group2  block_type=convert  block_config=sysgen:Convert_config  block_width=595  block_height=885
  Convert8 : hdlBasic/Convert  gui_display_data_type=Fixed-point  arith_type="Signed  (2's comp)"  n_bits=17  bin_pt=16  float_type=Single  exp_bits=8  fraction_bits=24  quantization=Truncate  overflow=Saturate  en=off  latency=0  pipeline=off  XmcBlockStatus=1  maskContainerNames=group2  block_type=convert  block_config=sysgen:Convert_config  block_width=595  block_height=885
  Dual Port RAM1 A : hdlBasic/Simple Dual Port RAM  depth=ChirpNc*RXFFTLength  initVector=0  distributed_mem=Distributed memory  init_b=0  rst_b=off  en_a=on  en_b=off  latency=1  write_mode_B=Read After Write  explicit_period=[]  period=[]  simulation_type=fast_sim  XmcBlockStatus=1  maskContainerNames=tabcontainer1  block_type=sdpram  block_config=sysgen:Sdpram_config  optimize=Area
      settings: infoedit=[]
  Dual Port RAM1 B : hdlBasic/Simple Dual Port RAM  depth=ChirpNc*RXFFTLength  initVector=0  distributed_mem=Distributed memory  init_b=0  rst_b=off  en_a=on  en_b=off  latency=1  write_mode_B=Read After Write  explicit_period=[]  period=[]  simulation_type=fast_sim  XmcBlockStatus=1  maskContainerNames=tabcontainer1  block_type=sdpram  block_config=sysgen:Sdpram_config  optimize=Area
      settings: infoedit=[]
  Dual Port RAM2 A : hdlBasic/Simple Dual Port RAM  depth=ChirpNc*RXFFTLength  initVector=0  distributed_mem=Distributed memory  init_b=0  rst_b=off  en_a=on  en_b=off  latency=1  write_mode_B=Read After Write  explicit_period=[]  period=[]  simulation_type=fast_sim  XmcBlockStatus=1  maskContainerNames=tabcontainer1  block_type=sdpram  block_config=sysgen:Sdpram_config  optimize=Area
      settings: infoedit=[]
  Dual Port RAM2 B : hdlBasic/Simple Dual Port RAM  depth=ChirpNc*RXFFTLength  initVector=0  distributed_mem=Distributed memory  init_b=0  rst_b=off  en_a=on  en_b=off  latency=1  write_mode_B=Read After Write  explicit_period=[]  period=[]  simulation_type=fast_sim  XmcBlockStatus=1  maskContainerNames=tabcontainer1  block_type=sdpram  block_config=sysgen:Sdpram_config  optimize=Area
      settings: infoedit=[]
  DualRAMOutSW1 : hdlBasic/Mux  inputs=2  en=off  latency=0  precision=Full  arith_type=Unsigned  n_bits=16  bin_pt=14  quantization=Truncate  overflow=Wrap  XmcBlockStatus=1  maskContainerNames=tabcontainer1  block_type=mux  block_config=sysgen:Mux_config
  DualRAMOutSW2 : hdlBasic/Mux  inputs=2  en=off  latency=0  precision=Full  arith_type=Unsigned  n_bits=16  bin_pt=14  quantization=Truncate  overflow=Wrap  XmcBlockStatus=1  maskContainerNames=tabcontainer1  block_type=mux  block_config=sysgen:Mux_config
  Inverter1 : hdlBasic/Inverter  en=off  latency=0  XmcBlockStatus=1  maskContainerNames=group2  block_type=inv  block_config=sysgen:Inverter_config
  Mux12 : hdlBasic/Mux  inputs=2  en=off  latency=0  precision=Full  arith_type=Unsigned  n_bits=16  bin_pt=14  quantization=Truncate  overflow=Wrap  XmcBlockStatus=1  maskContainerNames=tabcontainer1  block_type=mux  block_config=sysgen:Mux_config
  Mux13 : hdlBasic/Mux  inputs=2  en=off  latency=0  precision=Full  arith_type=Unsigned  n_bits=16  bin_pt=14  quantization=Truncate  overflow=Wrap  XmcBlockStatus=1  maskContainerNames=tabcontainer1  block_type=mux  block_config=sysgen:Mux_config
  Null1 : hdlBasic/Constant  const=0  gui_display_data_type=Fixed-point  arith_type=Signed (2's comp)  n_bits=16  bin_pt=15  preci_type=Single  exp_width=8  frac_width=24  explicit_period=on  period=P2  XmcBlockStatus=1  maskContainerNames=tabcontainer1  block_type=constant  block_config=sysgen:Constant_config
  Null2 : hdlBasic/Constant  const=0  gui_display_data_type=Boolean  arith_type=Boolean  n_bits=16  bin_pt=15  preci_type=Single  exp_width=8  frac_width=24  explicit_period=on  period=P2  XmcBlockStatus=1  maskContainerNames=tabcontainer1  block_type=constant  block_config=sysgen:Constant_config
  WEDisEnbA : hdlBasic/Mux  inputs=2  en=off  latency=0  precision=Full  arith_type=Unsigned  n_bits=16  bin_pt=14  quantization=Truncate  overflow=Wrap  XmcBlockStatus=1  maskContainerNames=tabcontainer1  block_type=mux  block_config=sysgen:Mux_config
  WEDisEnbB : hdlBasic/Mux  inputs=2  en=off  latency=0  precision=Full  arith_type=Unsigned  n_bits=16  bin_pt=14  quantization=Truncate  overflow=Wrap  XmcBlockStatus=1  maskContainerNames=tabcontainer1  block_type=mux  block_config=sysgen:Mux_config
  RngRETx1 : Outport
  RngIMGTx1 : Outport  Port=2
  wires:
  Mux13/1 -> RngIMGTx1/1
  Mux12/1 -> RngRETx1/1
  Convert8/1 -> Mux13/3
  Convert7/1 -> Mux12/3
  TransmitSel/1 -> Mux12/1, Mux13/1
  Dual Port RAM2 A/1 -> DualRAMOutSW2/3
  Dual Port RAM1 A/1 -> DualRAMOutSW1/3
  Null1/1 -> Mux13/2, Mux12/2
  Dual Port RAM1 B/1 -> DualRAMOutSW1/2
  DualRAMOutSW1/1 -> Convert7/1
  DataRE/1 -> Dual Port RAM1 B/2, Dual Port RAM1 A/2
  DataIMG/1 -> Dual Port RAM2 B/2, Dual Port RAM2 A/2
  EN/1 -> Dual Port RAM1 A/5, Dual Port RAM1 B/5, Dual Port RAM2 B/5, Dual Port RAM2 A/5
  Null2/1 -> WEDisEnbB/3, WEDisEnbA/3
  Dual Port RAM2 B/1 -> DualRAMOutSW2/2
  DualRAMOutSW2/1 -> Convert8/1
  WE/1 -> WEDisEnbB/2, WEDisEnbA/2
  AddressA/1 -> Dual Port RAM1 A/1, Dual Port RAM1 B/1, Dual Port RAM2 A/1, Dual Port RAM2 B/1
  AddressB/1 -> Dual Port RAM2 A/4, Dual Port RAM2 B/4, Dual Port RAM1 B/4, Dual Port RAM1 A/4
  Inverter1/1 -> WEDisEnbB/1
  SwapRAM/1 -> Inverter1/1, WEDisEnbA/1, DualRAMOutSW2/1, DualRAMOutSW1/1
  WEDisEnbA/1 -> Dual Port RAM2 A/3, Dual Port RAM1 A/3
  WEDisEnbB/1 -> Dual Port RAM2 B/3, Dual Port RAM1 B/3

== system RadarSimulinkProjectRev009/RangeProcessing/FFTTracking ==
  note: Should restart counter at beggining or end,
      | In Radix mode, Tlast is not the beggining because there is a gap
  note: In Radix burst, this is active for only real frame of data
      | In Pipeline, it's always active
  note: Bring back to 0 at start
  note: Only count for valid FFT points of data
      | Note: Add reset later
  data_Active : Inport
  StatusReady : Inport  Port=2
  DecimatedTrig : Inport  Port=3
  AddrforIQvals : hdlBasic/Counter  cnt_type=Count limited  cnt_to=ChirpNc*RXFFTLength-1  operation=Up  start_count=0  cnt_by_val=1  arith_type=Unsigned  n_bits=18  bin_pt=0  load_pin=off  rst=off  en=on  explicit_period=Explicit  period=P1  use_behavioral_HDL=off  implementation=Fabric  XmcBlockStatus=1  maskContainerNames=group1  block_type=counter  block_config=sysgen:Counter_config  block_width=531  block_height=1023
  Gateway Out1 : hdlBasic/Gateway Out  inherit_from_input=off  bool_to_boolean=off  hdl_port=on  rows=1  columns=1  UseAsDAC=off  DACChannel='1'  interface=None  automatic_assignment=on  address_offset=hex2dec('00')  intf_name=''  intf_description=''  timing_constraint=None  locs_specified=off  LOCs={}  io_standard={}  XmcBlockStatus=1  maskContainerNames=group4  block_type=gatewayout  block_config=sysgen:gateway_out_config  block_width_w=590  block_height_w=620  block_width=620  block_height=750
  Gateway Out15 : hdlBasic/Gateway Out  inherit_from_input=off  bool_to_boolean=off  hdl_port=on  rows=1  columns=1  UseAsDAC=off  DACChannel='1'  interface=None  automatic_assignment=on  address_offset=hex2dec('00')  intf_name=''  intf_description=''  timing_constraint=None  locs_specified=off  LOCs={}  io_standard={}  XmcBlockStatus=1  maskContainerNames=group4  block_type=gatewayout  block_config=sysgen:gateway_out_config  block_width_w=590  block_height_w=620  block_width=620  block_height=750
  Gateway Out4 : hdlBasic/Gateway Out  inherit_from_input=off  bool_to_boolean=off  hdl_port=on  rows=1  columns=1  UseAsDAC=off  DACChannel='1'  interface=None  automatic_assignment=on  address_offset=hex2dec('00')  intf_name=''  intf_description=''  timing_constraint=None  locs_specified=off  LOCs={}  io_standard={}  XmcBlockStatus=1  maskContainerNames=group4  block_type=gatewayout  block_config=sysgen:gateway_out_config  block_width_w=590  block_height_w=620  block_width=620  block_height=750
  IndexTracker : hdlBasic/Counter  cnt_type=Count limited  cnt_to=RXFFTLength*DeciFactor-1  operation=Up  start_count=0  cnt_by_val=1  arith_type=Unsigned  n_bits=14  bin_pt=0  load_pin=off  rst=on  en=on  explicit_period=Explicit  period=P1  use_behavioral_HDL=off  implementation=Fabric  XmcBlockStatus=1  maskContainerNames=group1  block_type=counter  block_config=sysgen:Counter_config  block_width=531  block_height=1023
  Inverter : hdlBasic/Inverter  en=off  latency=0  XmcBlockStatus=1  maskContainerNames=group2  block_type=inv  block_config=sysgen:Inverter_config
  Logical1 : hdlBasic/Logical  logical_function=AND  inputs=2  en=off  latency=0  precision=Full  arith_type=Unsigned  n_bits=16  bin_pt=0  align_bp=on  overflow=[]  quantization=[]  XmcBlockStatus=1  maskContainerNames=tabcontainer1  block_type=logical  block_config=sysgen:Logical_config
  Logical2 : hdlBasic/Logical  logical_function=AND  inputs=2  en=off  latency=0  precision=Full  arith_type=Unsigned  n_bits=16  bin_pt=0  align_bp=on  overflow=[]  quantization=[]  XmcBlockStatus=1  maskContainerNames=tabcontainer1  block_type=logical  block_config=sysgen:Logical_config
  Scope3 : Scope  NumInputPorts=3
  FFTIndex : Outport
  PeakSerachEnable : Outport  Port=2
  IQDataADDR : Outport  Port=3
  wires:
  IndexTracker/1 -> FFTIndex/1
  Inverter/1 -> IndexTracker/1
  DecimatedTrig/1 -> Gateway Out15/1, Logical2/1
  Logical1/1 -> PeakSerachEnable/1, IndexTracker/2
  StatusReady/1 -> Logical1/1, Inverter/1
  data_Active/1 -> Logical2/2, Logical1/2
  AddrforIQvals/1 -> Gateway Out1/1, IQDataADDR/1
  Logical2/1 -> Gateway Out4/1, AddrforIQvals/1
  Gateway Out15/1 -> Scope3/3
  Gateway Out1/1 -> Scope3/2
  Gateway Out4/1 -> Scope3/1

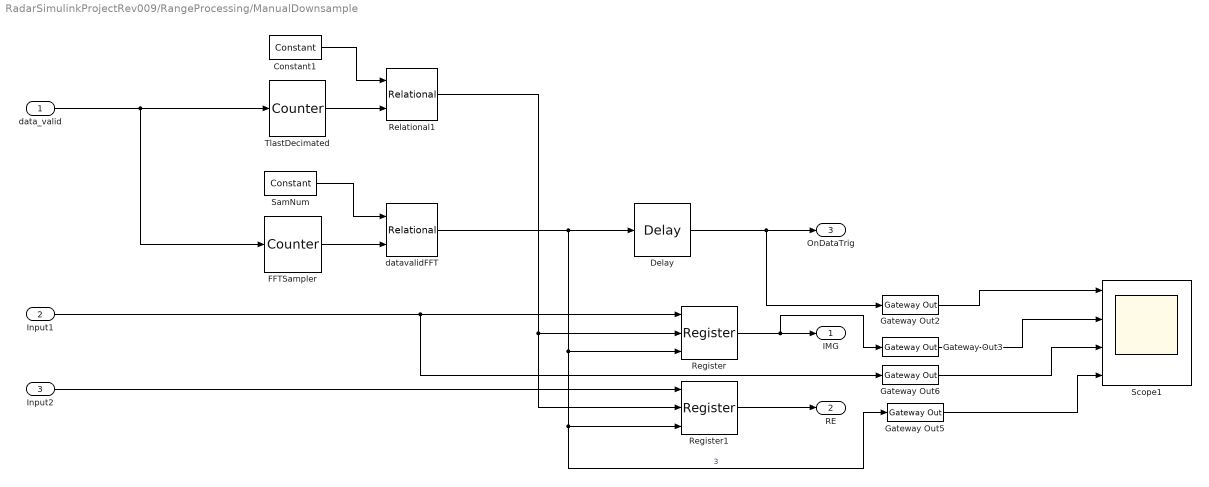
== system RadarSimulinkProjectRev009/RangeProcessing/ManualDownsample ==
  data_valid : Inport
  Input1 : Inport  Port=2
  Input2 : Inport  Port=3
  Constant1 : hdlBasic/Constant  const=RXFFTLength*8-1  gui_display_data_type=Fixed-point  arith_type=Signed (2's comp)  n_bits=16  bin_pt=0  preci_type=Single  exp_width=8  frac_width=24  explicit_period=off  period=1  XmcBlockStatus=1  maskContainerNames=tabcontainer1  block_type=constant  block_config=sysgen:Constant_config
  Delay : hdlBasic/Delay  rst=off  en=off  latency=1  reg_retiming=off  XmcBlockStatus=1  maskContainerNames=group1  block_type=delay  block_config=sysgen:Delay_config
  FFTSampler : hdlBasic/Counter  cnt_type=Count limited  cnt_to=DeciFactor-1  operation=Up  start_count=0  cnt_by_val=1  arith_type=Unsigned  n_bits=4  bin_pt=0  load_pin=off  rst=off  en=on  explicit_period=Explicit  period=P1  use_behavioral_HDL=off  implementation=Fabric  XmcBlockStatus=1  maskContainerNames=group1  block_type=counter  block_config=sysgen:Counter_config  block_width=531  block_height=1023
  Gateway Out{2..3,5..6} (4 alike) : hdlBasic/Gateway Out  inherit_from_input=off  bool_to_boolean=off  hdl_port=on  rows=1  columns=1  UseAsDAC=off  DACChannel='1'  interface=None  automatic_assignment=on  address_offset=hex2dec('00')  intf_name=''  intf_description=''  timing_constraint=None  locs_specified=off  LOCs={}  io_standard={}  XmcBlockStatus=1  maskContainerNames=group4  block_type=gatewayout  block_config=sysgen:gateway_out_config  block_width_w=590  block_height_w=620  block_width=620  block_height=750
  Register : hdlBasic/Register  init=0  rst=on  en=on  XmcBlockStatus=1  maskContainerNames=tabcontainer1  block_type=register  block_config=sysgen:Register_config
  Register1 : hdlBasic/Register  init=0  rst=on  en=on  XmcBlockStatus=1  maskContainerNames=tabcontainer1  block_type=register  block_config=sysgen:Register_config
  Relational1 : hdlBasic/Relational  mode=a=b  op_type=Bool  en=off  latency=0  XmcBlockStatus=1  maskContainerNames=tabcontainer1  block_type=relational  block_config=sysgen:Relational_config
  SamNum : hdlBasic/Constant  const=0  gui_display_data_type=Fixed-point  arith_type=Signed (2's comp)  n_bits=5  bin_pt=0  preci_type=Single  exp_width=8  frac_width=24  explicit_period=off  period=1  XmcBlockStatus=1  maskContainerNames=tabcontainer1  block_type=constant  block_config=sysgen:Constant_config
  Scope1 : Scope  NumInputPorts=4
  TlastDecimated : hdlBasic/Counter  cnt_type=Count limited  cnt_to=2047  operation=Up  start_count=0  cnt_by_val=1  arith_type=Unsigned  n_bits=12  bin_pt=0  load_pin=off  rst=off  en=on  explicit_period=Inferred from inputs  period=P1  use_behavioral_HDL=off  implementation=Fabric  XmcBlockStatus=1  maskContainerNames=group1  block_type=counter  block_config=sysgen:Counter_config  block_width=531  block_height=1023
  datavalidFFT : hdlBasic/Relational  mode=a=b  op_type=Bool  en=off  latency=0  XmcBlockStatus=1  maskContainerNames=tabcontainer1  block_type=relational  block_config=sysgen:Relational_config
  IMG : Outport
  RE : Outport  Port=2
  OnDataTrig : Outport  Port=3
  wires:
  data_valid/1 -> FFTSampler/1, TlastDecimated/1
  Constant1/1 -> Relational1/1
  FFTSampler/1 -> datavalidFFT/2
  datavalidFFT/1 -> Gateway Out5/1, Register1/3, Register/3, Delay/1  "3"
  TlastDecimated/1 -> Relational1/2
  SamNum/1 -> datavalidFFT/1
  Register/1 -> Gateway Out3/1, IMG/1
  Register1/1 -> RE/1
  Delay/1 -> Gateway Out2/1, OnDataTrig/1
  Input1/1 -> Gateway Out6/1, Register/1
  Input2/1 -> Register1/1
  Relational1/1 -> Register/2, Register1/2
  Gateway Out3/1 -> Scope1/2
  Gateway Out6/1 -> Scope1/3
  Gateway Out5/1 -> Scope1/4
  Gateway Out2/1 -> Scope1/1
